simulink model "LDR"  (R2024a)
settings: Solver=FixedStepDiscrete  StartTime=0.0  StopTime=10.0  FixedStep=.01  RelTol=1e-3
settings Model: Creator=User  LastModifiedBy=User
settings OptimizationCC: DefaultParameterBehavior=Inlined  UseDivisionForNetSlopeComputation=on  GainParamInheritBuiltInType=on  UseFloatMulNetSlope=on  InlineInvariantSignals=on  PassReuseOutputArgsAs=Individual arguments  ZeroExternalMemoryAtStartup=off  ZeroInternalMemoryAtStartup=off  NoFixptDivByZeroProtection=on  EfficientFloat2IntCast=on  LifeSpan=1  OptimizeBlockOrder=speed  DifferentSizesBufferReuse=on  EfficientTunableParamExpr=on
settings DebuggingCC: ParameterTunabilityLossMsg=error
settings HardwareCC: ProdBitPerInt=16  ProdBitPerPointer=16  ProdBitPerSizeT=16  ProdBitPerPtrDiffT=16  ProdLargestAtomicFloat=None  ProdWordSize=16  ProdLongLongMode=on  ProdHWDeviceType=Atmel->AVR (8-bit)
settings SFSimCC: MATLABDynamicMemAlloc=off
settings RTWCC: Description=Embedded Coder  SystemTargetFile=ert.tlc  GenCodeOnly=on  TemplateMakefile=ert_default_tmf  GenerateReport=on  LaunchReport=on  GenerateCodeMetricsReport=on
settings CodeAppCC: ForceParamTrailComments=on  IgnoreCustomStorageClasses=off  OperatorAnnotations=on  SimulinkDataObjDesc=on  SFDataObjDesc=on  CustomSymbolStrGlobalVar=rt$N$M  CustomSymbolStrType=$N$M  CustomSymbolStrFcn=$N$M$F  CustomSymbolStrMacro=$N$M  InsertBlockDesc=on
settings ERTTargetCC: TargetLangStandard=C99 (ISO)  GenerateSampleERTMain=on  IncludeMdlTerminateFcn=off  CombineSignalStateStructs=on  SuppressErrorStatus=on  SupportAbsoluteTime=off  PurelyIntegerCode=on  SupportNonFinite=off  SupportComplex=off  InlinedParameterPlacement=NonHierarchical  ERTCustomFileTemplate=example_file_process.tlc

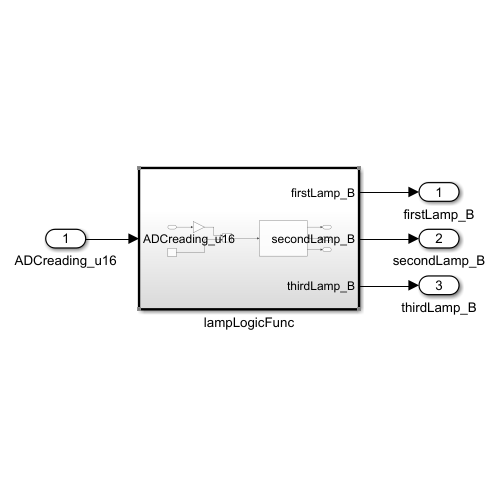
[thumbnail: Simulink's stored preview of the top-level diagram]
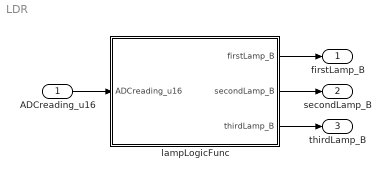
== system LDR ==
  ADCreading_u16 : Inport  OutDataTypeStr=uint16
  lampLogicFunc : Subsystem  TreatAsAtomicUnit=on
      settings: RTWFcnNameOpts=Use subsystem name  RTWFileNameOpts=Use subsystem name
  firstLamp_B : Outport  OutDataTypeStr=boolean
  secondLamp_B : Outport  Port=2  OutDataTypeStr=boolean
  thirdLamp_B : Outport  Port=3  OutDataTypeStr=boolean
  wires:
  ADCreading_u16/1 -> lampLogicFunc/1(ADCreading_u16)
  lampLogicFunc/1(firstLamp_B) -> firstLamp_B/1
  lampLogicFunc/2(secondLamp_B) -> secondLamp_B/1
  lampLogicFunc/3(thirdLamp_B) -> thirdLamp_B/1

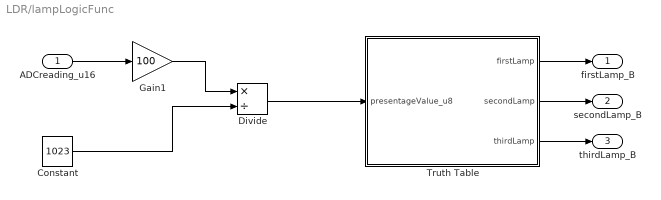
== system LDR/lampLogicFunc ==
  ADCreading_u16 : Inport  OutDataTypeStr=uint16
  Constant : Constant  Value=1023  OutDataTypeStr=uint16
  Divide : Product  Inputs=*/  OutDataTypeStr=uint8
  Gain1 : Gain  Gain=100  OutDataTypeStr=uint32
  Truth Table : Truth Table  TreatAsAtomicUnit=on
  firstLamp_B : Outport  OutDataTypeStr=boolean
  secondLamp_B : Outport  Port=2  OutDataTypeStr=boolean
  thirdLamp_B : Outport  Port=3  OutDataTypeStr=boolean
  wires:
  Divide/1 -> Truth Table/1(presentageValue_u8)
  Truth Table/1(firstLamp) -> firstLamp_B/1
  Truth Table/2(secondLamp) -> secondLamp_B/1
  Truth Table/3(thirdLamp) -> thirdLamp_B/1
  ADCreading_u16/1 -> Gain1/1
  Constant/1 -> Divide/2
  Gain1/1 -> Divide/1

== matlab function LDR/lampLogicFunc/Truth Table ==
  data: presentageValue_u8 input uint8; firstLamp output boolean; secondLamp output boolean; thirdLamp output boolean
function [firstLamp, secondLamp, thirdLamp] = fcn(presentageValue_u8)

aVarTruthTableCondition_1 = false;
aVarTruthTableCondition_2 = false;
aVarTruthTableCondition_3 = false;


% Example condition 1

aVarTruthTableCondition_1 = logical(presentageValue_u8>60);

% Example condition 2

aVarTruthTableCondition_2 = logical(presentageValue_u8>40);

% Condition #3
aVarTruthTableCondition_3 = logical(presentageValue_u8>20);

if (aVarTruthTableCondition_1)
    aFcnTruthTableAction_1();
elseif (aVarTruthTableCondition_2)
    aFcnTruthTableAction_2();
elseif (aVarTruthTableCondition_3)
    aFcnTruthTableAction_3();
else % Default
    aFcnTruthTableAction_4();
end

function aFcnTruthTableAction_1()

% Example action 1 called from D1 & D2 column in condition table

firstLamp =true;
secondLamp=true;
thirdLamp=true;

function aFcnTruthTableAction_2()



firstLamp =true;
secondLamp=true;
thirdLamp=false;

function aFcnTruthTableAction_3()

% Example action 2 called from D3 column in condition table

firstLamp =true;
secondLamp=false;
thirdLamp=false;

function aFcnTruthTableAction_4()



firstLamp =false;
secondLamp=false;
thirdLamp=false;
